simulink model "architecture_model"  (R2024a)
settings: Solver=VariableStepAuto  StartTime=0.0  StopTime=10.0  RelTol=1e-3
settings Model: Creator=nicol  LastModifiedBy=nicol

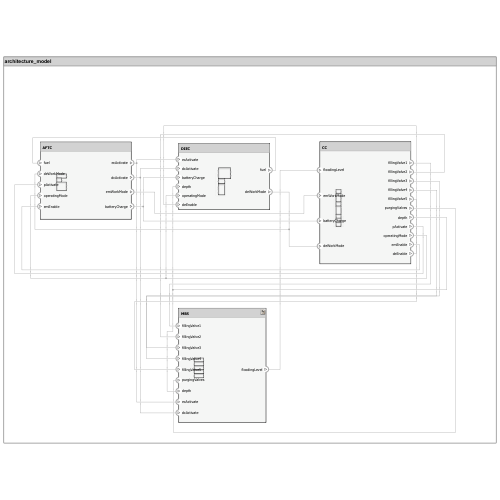
[thumbnail: Simulink's stored preview of the top-level diagram]
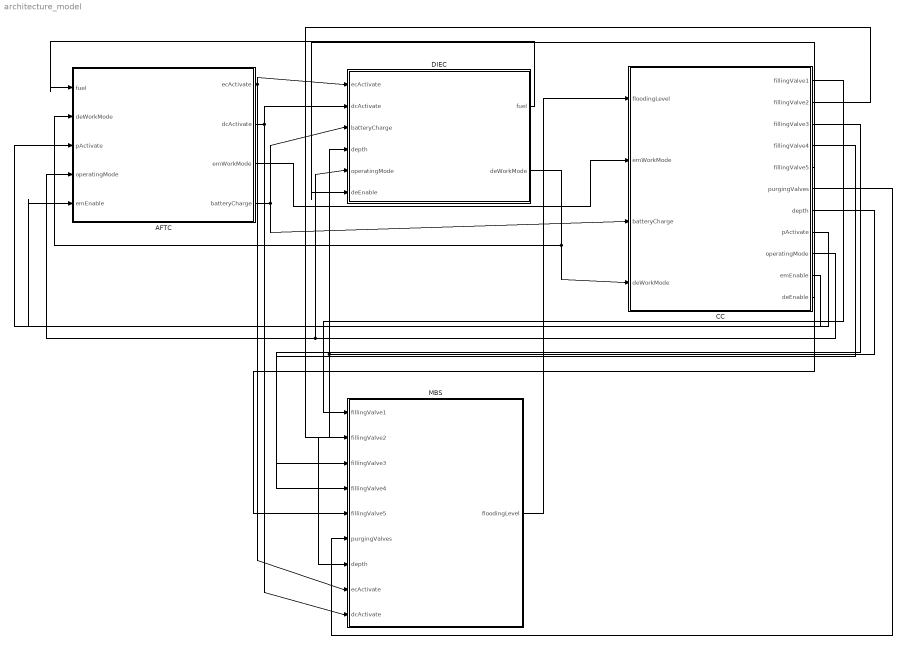
== system architecture_model ==
  AFTC : Subsystem
      settings: PortSchema="{\"entries\":[{\"content\":{\"headerSize\":26,\"margin\":15,\"minimumSpacing\":25,\"sides\":[{\"content\":{\"connectorIds\":[\"In1\",\"In2\",\"In3\",\"In4\",\"In5\"]},\"type\":\"ConnectorPlacement.EquallySpacedRectSide\",\"uuid\":\"054348e9-4623-4d1e-a130-1e3dd56bb1c6\"},{\"content\":{\"connectorIds\":[\"Out1\",\"Out2\",\"Out3\",\"Out4\"],\"side\":\"RIGHT\"},\"type\":\"ConnectorPlacement.EquallySpacedRectSide\",\"uuid\":\"04ca0bbb-2ad8-4415-8a15-39e786354471\"},{\"content\":{\"side\":\"TOP\"},\"type\":\"ConnectorPlacement.EquallySpacedRectSide\",\"uuid\":\"67b55d8f-8342-4ecc-881d-538334cee7ba\"}]},\"type\":\"ConnectorPlacement.EquallySpacedConnector\",\"uuid\":\"5f8a1871-b485-48ba-829b-ead526173e4c\"}],\"packageUris\":[\"http://schema.mathworks.com/mf0/Connector/R2020b\"],\"version\":\"1.0\"}"
  CC : Subsystem
      settings: PortSchema="{\"entries\":[{\"content\":{\"headerSize\":26,\"margin\":15,\"minimumSpacing\":25,\"sides\":[{\"content\":{\"connectorIds\":[\"In1\",\"In2\",\"In3\",\"In4\"]},\"type\":\"ConnectorPlacement.EquallySpacedRectSide\",\"uuid\":\"054348e9-4623-4d1e-a130-1e3dd56bb1c6\"},{\"content\":{\"connectorIds\":[\"Out1\",\"Out2\",\"Out3\",\"Out4\",\"Out5\",\"Out6\",\"Out7\",\"Out8\",\"Out9\",\"Out10\",\"Out11\"],\"side\":\"RIGHT\"},\"type\":\"ConnectorPlacement.EquallySpacedRectSide\",\"uuid\":\"04ca0bbb-2ad8-4415-8a15-39e786354471\"},{\"content\":{\"side\":\"TOP\"},\"type\":\"ConnectorPlacement.EquallySpacedRectSide\",\"uuid\":\"67b55d8f-8342-4ecc-881d-538334cee7ba\"}]},\"type\":\"ConnectorPlacement.EquallySpacedConnector\",\"uuid\":\"5f8a1871-b485-48ba-829b-ead526173e4c\"}],\"packageUris\":[\"http://schema.mathworks.com/mf0/Connector/R2020b\"],\"version\":\"1.0\"}"
  DIEC : Subsystem
      settings: PortSchema="{\"entries\":[{\"content\":{\"headerSize\":26,\"margin\":15,\"minimumSpacing\":25,\"sides\":[{\"content\":{\"connectorIds\":[\"In1\",\"In2\",\"In3\",\"In4\",\"In5\",\"In6\"]},\"type\":\"ConnectorPlacement.EquallySpacedRectSide\",\"uuid\":\"054348e9-4623-4d1e-a130-1e3dd56bb1c6\"},{\"content\":{\"connectorIds\":[\"Out1\",\"Out2\"],\"side\":\"RIGHT\"},\"type\":\"ConnectorPlacement.EquallySpacedRectSide\",\"uuid\":\"04ca0bbb-2ad8-4415-8a15-39e786354471\"},{\"content\":{\"side\":\"TOP\"},\"type\":\"ConnectorPlacement.EquallySpacedRectSide\",\"uuid\":\"67b55d8f-8342-4ecc-881d-538334cee7ba\"}]},\"type\":\"ConnectorPlacement.EquallySpacedConnector\",\"uuid\":\"5f8a1871-b485-48ba-829b-ead526173e4c\"}],\"packageUris\":[\"http://schema.mathworks.com/mf0/Connector/R2020b\"],\"version\":\"1.0\"}"
  MBS : Subsystem
      settings: PortSchema="{\"entries\":[{\"content\":{\"headerSize\":26,\"margin\":15,\"minimumSpacing\":25,\"sides\":[{\"content\":{\"connectorIds\":[\"In1\",\"In2\",\"In3\",\"In4\",\"In5\",\"In6\",\"In7\",\"In8\",\"In9\"]},\"type\":\"ConnectorPlacement.EquallySpacedRectSide\",\"uuid\":\"054348e9-4623-4d1e-a130-1e3dd56bb1c6\"},{\"content\":{\"connectorIds\":[\"Out1\"],\"side\":\"RIGHT\"},\"type\":\"ConnectorPlacement.EquallySpacedRectSide\",\"uuid\":\"04ca0bbb-2ad8-4415-8a15-39e786354471\"},{\"content\":{\"side\":\"TOP\"},\"type\":\"ConnectorPlacement.EquallySpacedRectSide\",\"uuid\":\"67b55d8f-8342-4ecc-881d-538334cee7ba\"}]},\"type\":\"ConnectorPlacement.EquallySpacedConnector\",\"uuid\":\"5f8a1871-b485-48ba-829b-ead526173e4c\"}],\"packageUris\":[\"http://schema.mathworks.com/mf0/Connector/R2020b\"],\"version\":\"1.0\"}"
  wires:
  AFTC/1(ecActivate) -> DIEC/1(ecActivate), MBS/8(ecActivate)
  MBS/1(floodingLevel) -> CC/1(floodingLevel)
  CC/1(fillingValve1) -> MBS/1(fillingValve1)
  CC/2(fillingValve2) -> MBS/2(fillingValve2)
  CC/3(fillingValve3) -> MBS/3(fillingValve3)
  CC/4(fillingValve4) -> MBS/4(fillingValve4)
  CC/5(fillingValve5) -> MBS/5(fillingValve5)
  CC/6(purgingValves) -> MBS/6(purgingValves)
  AFTC/2(dcActivate) -> DIEC/2(dcActivate), MBS/9(dcActivate)
  CC/7(depth) -> DIEC/4(depth), MBS/7(depth)
  DIEC/1(fuel) -> AFTC/1(fuel)
  AFTC/3(emWorkMode) -> CC/2(emWorkMode)
  AFTC/4(batteryCharge) -> DIEC/3(batteryCharge), CC/3(batteryCharge)
  DIEC/2(deWorkMode) -> AFTC/2(deWorkMode), CC/4(deWorkMode)
  CC/8(pActivate) -> AFTC/3(pActivate)
  CC/9(operatingMode) -> DIEC/5(operatingMode), AFTC/4(operatingMode)
  CC/10(emEnable) -> AFTC/5(emEnable)
  CC/11(deEnable) -> DIEC/6(deEnable)

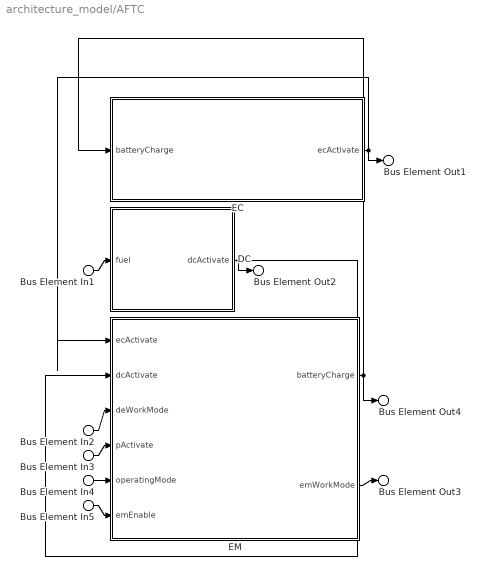
== system architecture_model/AFTC ==
  Bus Element In1 : Inport  PortName=fuel
  Bus Element In2 : Inport  Port=2  PortName=deWorkMode
  Bus Element In3 : Inport  Port=3  PortName=pActivate
  Bus Element In4 : Inport  Port=4  PortName=operatingMode
  Bus Element In5 : Inport  Port=5  PortName=emEnable
  DC : Subsystem
      settings: PortSchema="{\"entries\":[{\"content\":{\"headerSize\":26,\"margin\":15,\"minimumSpacing\":25,\"sides\":[{\"content\":{\"connectorIds\":[\"In1\"]},\"type\":\"ConnectorPlacement.EquallySpacedRectSide\",\"uuid\":\"054348e9-4623-4d1e-a130-1e3dd56bb1c6\"},{\"content\":{\"connectorIds\":[\"Out1\"],\"side\":\"RIGHT\"},\"type\":\"ConnectorPlacement.EquallySpacedRectSide\",\"uuid\":\"04ca0bbb-2ad8-4415-8a15-39e786354471\"},{\"content\":{\"side\":\"TOP\"},\"type\":\"ConnectorPlacement.EquallySpacedRectSide\",\"uuid\":\"67b55d8f-8342-4ecc-881d-538334cee7ba\"}]},\"type\":\"ConnectorPlacement.EquallySpacedConnector\",\"uuid\":\"5f8a1871-b485-48ba-829b-ead526173e4c\"}],\"packageUris\":[\"http://schema.mathworks.com/mf0/Connector/R2020b\"],\"version\":\"1.0\"}"
  EC : Subsystem
      settings: PortSchema="{\"entries\":[{\"content\":{\"headerSize\":26,\"margin\":15,\"minimumSpacing\":25,\"sides\":[{\"content\":{\"connectorIds\":[\"In1\"]},\"type\":\"ConnectorPlacement.EquallySpacedRectSide\",\"uuid\":\"054348e9-4623-4d1e-a130-1e3dd56bb1c6\"},{\"content\":{\"connectorIds\":[\"Out1\"],\"side\":\"RIGHT\"},\"type\":\"ConnectorPlacement.EquallySpacedRectSide\",\"uuid\":\"04ca0bbb-2ad8-4415-8a15-39e786354471\"},{\"content\":{\"side\":\"TOP\"},\"type\":\"ConnectorPlacement.EquallySpacedRectSide\",\"uuid\":\"67b55d8f-8342-4ecc-881d-538334cee7ba\"}]},\"type\":\"ConnectorPlacement.EquallySpacedConnector\",\"uuid\":\"5f8a1871-b485-48ba-829b-ead526173e4c\"}],\"packageUris\":[\"http://schema.mathworks.com/mf0/Connector/R2020b\"],\"version\":\"1.0\"}"
  EM : Subsystem
      settings: PortSchema="{\"entries\":[{\"content\":{\"headerSize\":26,\"margin\":15,\"minimumSpacing\":25,\"sides\":[{\"content\":{\"connectorIds\":[\"In1\",\"In2\",\"In3\",\"In4\",\"In5\",\"In6\"]},\"type\":\"ConnectorPlacement.EquallySpacedRectSide\",\"uuid\":\"054348e9-4623-4d1e-a130-1e3dd56bb1c6\"},{\"content\":{\"connectorIds\":[\"Out1\",\"Out2\"],\"side\":\"RIGHT\"},\"type\":\"ConnectorPlacement.EquallySpacedRectSide\",\"uuid\":\"04ca0bbb-2ad8-4415-8a15-39e786354471\"},{\"content\":{\"side\":\"TOP\"},\"type\":\"ConnectorPlacement.EquallySpacedRectSide\",\"uuid\":\"67b55d8f-8342-4ecc-881d-538334cee7ba\"}]},\"type\":\"ConnectorPlacement.EquallySpacedConnector\",\"uuid\":\"5f8a1871-b485-48ba-829b-ead526173e4c\"}],\"packageUris\":[\"http://schema.mathworks.com/mf0/Connector/R2020b\"],\"version\":\"1.0\"}"
  Bus Element Out1 : Outport  PortName=ecActivate
  Bus Element Out2 : Outport  Port=2  PortName=dcActivate
  Bus Element Out3 : Outport  Port=3  PortName=emWorkMode
  Bus Element Out4 : Outport  Port=4  PortName=batteryCharge
  wires:
  EC/1(ecActivate) -> Bus Element Out1/1, EM/1(ecActivate)
  EM/1(batteryCharge) -> Bus Element Out4/1, EC/1(batteryCharge)
  DC/1(dcActivate) -> Bus Element Out2/1, EM/2(dcActivate)
  Bus Element In1/1 -> DC/1(fuel)
  EM/2(emWorkMode) -> Bus Element Out3/1
  Bus Element In2/1 -> EM/3(deWorkMode)
  Bus Element In3/1 -> EM/4(pActivate)
  Bus Element In4/1 -> EM/5(operatingMode)
  Bus Element In5/1 -> EM/6(emEnable)

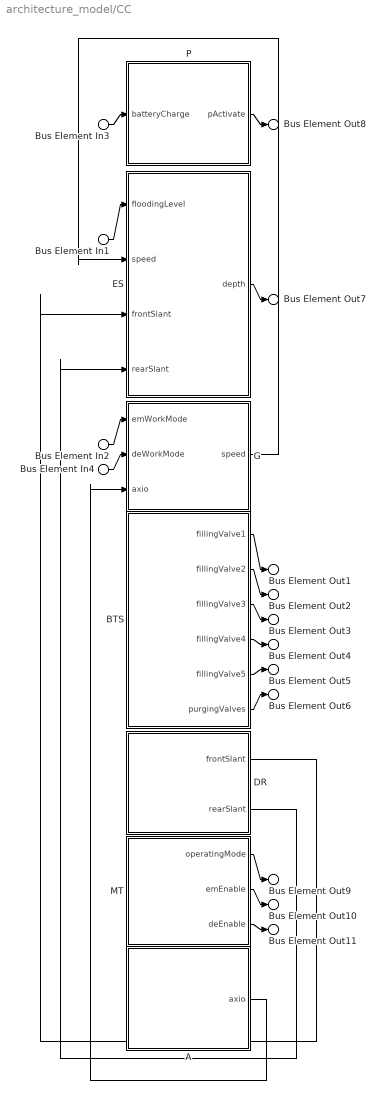
== system architecture_model/CC ==
  Bus Element In1 : Inport  PortName=floodingLevel
  Bus Element In2 : Inport  Port=2  PortName=emWorkMode
  Bus Element In3 : Inport  Port=3  PortName=batteryCharge
  Bus Element In4 : Inport  Port=4  PortName=deWorkMode
  A : Subsystem
      settings: PortSchema="{\"entries\":[{\"content\":{\"headerSize\":26,\"margin\":15,\"minimumSpacing\":25,\"sides\":[{\"content\":{},\"type\":\"ConnectorPlacement.EquallySpacedRectSide\",\"uuid\":\"054348e9-4623-4d1e-a130-1e3dd56bb1c6\"},{\"content\":{\"connectorIds\":[\"Out1\"],\"side\":\"RIGHT\"},\"type\":\"ConnectorPlacement.EquallySpacedRectSide\",\"uuid\":\"04ca0bbb-2ad8-4415-8a15-39e786354471\"},{\"content\":{\"side\":\"TOP\"},\"type\":\"ConnectorPlacement.EquallySpacedRectSide\",\"uuid\":\"67b55d8f-8342-4ecc-881d-538334cee7ba\"}]},\"type\":\"ConnectorPlacement.EquallySpacedConnector\",\"uuid\":\"5f8a1871-b485-48ba-829b-ead526173e4c\"}],\"packageUris\":[\"http://schema.mathworks.com/mf0/Connector/R2020b\"],\"version\":\"1.0\"}"
  BTS : Subsystem
      settings: PortSchema="{\"entries\":[{\"content\":{\"headerSize\":26,\"margin\":15,\"minimumSpacing\":25,\"sides\":[{\"content\":{},\"type\":\"ConnectorPlacement.EquallySpacedRectSide\",\"uuid\":\"054348e9-4623-4d1e-a130-1e3dd56bb1c6\"},{\"content\":{\"connectorIds\":[\"Out1\",\"Out2\",\"Out3\",\"Out4\",\"Out5\",\"Out6\"],\"side\":\"RIGHT\"},\"type\":\"ConnectorPlacement.EquallySpacedRectSide\",\"uuid\":\"04ca0bbb-2ad8-4415-8a15-39e786354471\"},{\"content\":{\"side\":\"TOP\"},\"type\":\"ConnectorPlacement.EquallySpacedRectSide\",\"uuid\":\"67b55d8f-8342-4ecc-881d-538334cee7ba\"}]},\"type\":\"ConnectorPlacement.EquallySpacedConnector\",\"uuid\":\"5f8a1871-b485-48ba-829b-ead526173e4c\"}],\"packageUris\":[\"http://schema.mathworks.com/mf0/Connector/R2020b\"],\"version\":\"1.0\"}"
  DR : Subsystem
      settings: PortSchema="{\"entries\":[{\"content\":{\"headerSize\":26,\"margin\":15,\"minimumSpacing\":25,\"sides\":[{\"content\":{},\"type\":\"ConnectorPlacement.EquallySpacedRectSide\",\"uuid\":\"054348e9-4623-4d1e-a130-1e3dd56bb1c6\"},{\"content\":{\"connectorIds\":[\"Out1\",\"Out2\"],\"side\":\"RIGHT\"},\"type\":\"ConnectorPlacement.EquallySpacedRectSide\",\"uuid\":\"04ca0bbb-2ad8-4415-8a15-39e786354471\"},{\"content\":{\"side\":\"TOP\"},\"type\":\"ConnectorPlacement.EquallySpacedRectSide\",\"uuid\":\"67b55d8f-8342-4ecc-881d-538334cee7ba\"}]},\"type\":\"ConnectorPlacement.EquallySpacedConnector\",\"uuid\":\"5f8a1871-b485-48ba-829b-ead526173e4c\"}],\"packageUris\":[\"http://schema.mathworks.com/mf0/Connector/R2020b\"],\"version\":\"1.0\"}"
  ES : Subsystem
      settings: PortSchema="{\"entries\":[{\"content\":{\"headerSize\":26,\"margin\":15,\"minimumSpacing\":25,\"sides\":[{\"content\":{\"connectorIds\":[\"In1\",\"In2\",\"In3\",\"In4\"]},\"type\":\"ConnectorPlacement.EquallySpacedRectSide\",\"uuid\":\"054348e9-4623-4d1e-a130-1e3dd56bb1c6\"},{\"content\":{\"connectorIds\":[\"Out1\"],\"side\":\"RIGHT\"},\"type\":\"ConnectorPlacement.EquallySpacedRectSide\",\"uuid\":\"04ca0bbb-2ad8-4415-8a15-39e786354471\"},{\"content\":{\"side\":\"TOP\"},\"type\":\"ConnectorPlacement.EquallySpacedRectSide\",\"uuid\":\"67b55d8f-8342-4ecc-881d-538334cee7ba\"}]},\"type\":\"ConnectorPlacement.EquallySpacedConnector\",\"uuid\":\"5f8a1871-b485-48ba-829b-ead526173e4c\"}],\"packageUris\":[\"http://schema.mathworks.com/mf0/Connector/R2020b\"],\"version\":\"1.0\"}"
  G : Subsystem
      settings: PortSchema="{\"entries\":[{\"content\":{\"headerSize\":26,\"margin\":15,\"minimumSpacing\":25,\"sides\":[{\"content\":{\"connectorIds\":[\"In1\",\"In2\",\"In3\"]},\"type\":\"ConnectorPlacement.EquallySpacedRectSide\",\"uuid\":\"054348e9-4623-4d1e-a130-1e3dd56bb1c6\"},{\"content\":{\"connectorIds\":[\"Out1\"],\"side\":\"RIGHT\"},\"type\":\"ConnectorPlacement.EquallySpacedRectSide\",\"uuid\":\"04ca0bbb-2ad8-4415-8a15-39e786354471\"},{\"content\":{\"side\":\"TOP\"},\"type\":\"ConnectorPlacement.EquallySpacedRectSide\",\"uuid\":\"67b55d8f-8342-4ecc-881d-538334cee7ba\"}]},\"type\":\"ConnectorPlacement.EquallySpacedConnector\",\"uuid\":\"5f8a1871-b485-48ba-829b-ead526173e4c\"}],\"packageUris\":[\"http://schema.mathworks.com/mf0/Connector/R2020b\"],\"version\":\"1.0\"}"
  MT : Subsystem
      settings: PortSchema="{\"entries\":[{\"content\":{\"headerSize\":26,\"margin\":15,\"minimumSpacing\":25,\"sides\":[{\"content\":{},\"type\":\"ConnectorPlacement.EquallySpacedRectSide\",\"uuid\":\"054348e9-4623-4d1e-a130-1e3dd56bb1c6\"},{\"content\":{\"connectorIds\":[\"Out1\",\"Out2\",\"Out3\"],\"side\":\"RIGHT\"},\"type\":\"ConnectorPlacement.EquallySpacedRectSide\",\"uuid\":\"04ca0bbb-2ad8-4415-8a15-39e786354471\"},{\"content\":{\"side\":\"TOP\"},\"type\":\"ConnectorPlacement.EquallySpacedRectSide\",\"uuid\":\"67b55d8f-8342-4ecc-881d-538334cee7ba\"}]},\"type\":\"ConnectorPlacement.EquallySpacedConnector\",\"uuid\":\"5f8a1871-b485-48ba-829b-ead526173e4c\"}],\"packageUris\":[\"http://schema.mathworks.com/mf0/Connector/R2020b\"],\"version\":\"1.0\"}"
  P : Subsystem
      settings: PortSchema="{\"entries\":[{\"content\":{\"headerSize\":26,\"margin\":15,\"minimumSpacing\":25,\"sides\":[{\"content\":{\"connectorIds\":[\"In1\"]},\"type\":\"ConnectorPlacement.EquallySpacedRectSide\",\"uuid\":\"054348e9-4623-4d1e-a130-1e3dd56bb1c6\"},{\"content\":{\"connectorIds\":[\"Out1\"],\"side\":\"RIGHT\"},\"type\":\"ConnectorPlacement.EquallySpacedRectSide\",\"uuid\":\"04ca0bbb-2ad8-4415-8a15-39e786354471\"},{\"content\":{\"side\":\"TOP\"},\"type\":\"ConnectorPlacement.EquallySpacedRectSide\",\"uuid\":\"67b55d8f-8342-4ecc-881d-538334cee7ba\"}]},\"type\":\"ConnectorPlacement.EquallySpacedConnector\",\"uuid\":\"5f8a1871-b485-48ba-829b-ead526173e4c\"}],\"packageUris\":[\"http://schema.mathworks.com/mf0/Connector/R2020b\"],\"version\":\"1.0\"}"
  Bus Element Out1 : Outport  PortName=fillingValve1
  Bus Element Out2 : Outport  Port=2  PortName=fillingValve2
  Bus Element Out3 : Outport  Port=3  PortName=fillingValve3
  Bus Element Out4 : Outport  Port=4  PortName=fillingValve4
  Bus Element Out5 : Outport  Port=5  PortName=fillingValve5
  Bus Element Out6 : Outport  Port=6  PortName=purgingValves
  Bus Element Out7 : Outport  Port=7  PortName=depth
  Bus Element Out8 : Outport  Port=8  PortName=pActivate
  Bus Element Out9 : Outport  Port=9  PortName=operatingMode
  Bus Element Out10 : Outport  Port=10  PortName=emEnable
  Bus Element Out11 : Outport  Port=11  PortName=deEnable
  wires:
  Bus Element In1/1 -> ES/1(floodingLevel)
  BTS/1(fillingValve1) -> Bus Element Out1/1
  BTS/2(fillingValve2) -> Bus Element Out2/1
  BTS/3(fillingValve3) -> Bus Element Out3/1
  BTS/4(fillingValve4) -> Bus Element Out4/1
  BTS/5(fillingValve5) -> Bus Element Out5/1
  BTS/6(purgingValves) -> Bus Element Out6/1
  ES/1(depth) -> Bus Element Out7/1
  Bus Element In2/1 -> G/1(emWorkMode)
  Bus Element In3/1 -> P/1(batteryCharge)
  P/1(pActivate) -> Bus Element Out8/1
  MT/1(operatingMode) -> Bus Element Out9/1
  MT/2(emEnable) -> Bus Element Out10/1
  Bus Element In4/1 -> G/2(deWorkMode)
  G/1(speed) -> ES/2(speed)
  DR/1(frontSlant) -> ES/3(frontSlant)
  DR/2(rearSlant) -> ES/4(rearSlant)
  A/1(axio) -> G/3(axio)
  MT/3(deEnable) -> Bus Element Out11/1

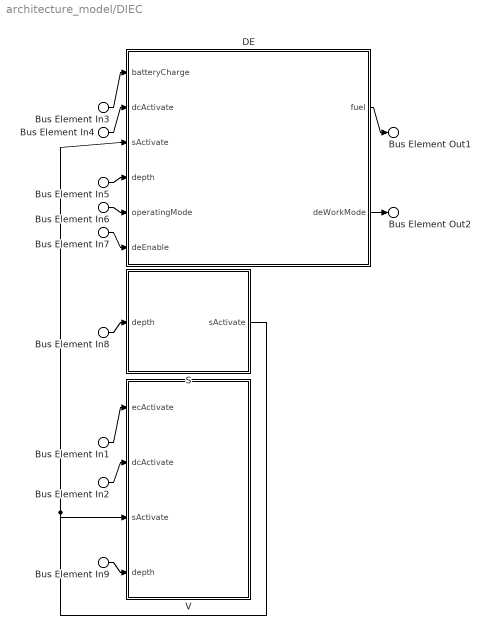
== system architecture_model/DIEC ==
  Bus Element In1 : Inport  PortName=ecActivate
  Bus Element In2 : Inport  Port=2  PortName=dcActivate
  Bus Element In4 : Inport  Port=2  PortName=dcActivate
  Bus Element In3 : Inport  Port=3  PortName=batteryCharge
  Bus Element In5 : Inport  Port=4  PortName=depth
  Bus Element In8 : Inport  Port=4  PortName=depth
  Bus Element In9 : Inport  Port=4  PortName=depth
  Bus Element In6 : Inport  Port=5  PortName=operatingMode
  Bus Element In7 : Inport  Port=6  PortName=deEnable
  DE : Subsystem
      settings: PortSchema="{\"entries\":[{\"content\":{\"headerSize\":26,\"margin\":15,\"minimumSpacing\":25,\"sides\":[{\"content\":{\"connectorIds\":[\"In1\",\"In2\",\"In3\",\"In4\",\"In5\",\"In6\"]},\"type\":\"ConnectorPlacement.EquallySpacedRectSide\",\"uuid\":\"054348e9-4623-4d1e-a130-1e3dd56bb1c6\"},{\"content\":{\"connectorIds\":[\"Out1\",\"Out2\"],\"side\":\"RIGHT\"},\"type\":\"ConnectorPlacement.EquallySpacedRectSide\",\"uuid\":\"04ca0bbb-2ad8-4415-8a15-39e786354471\"},{\"content\":{\"side\":\"TOP\"},\"type\":\"ConnectorPlacement.EquallySpacedRectSide\",\"uuid\":\"67b55d8f-8342-4ecc-881d-538334cee7ba\"}]},\"type\":\"ConnectorPlacement.EquallySpacedConnector\",\"uuid\":\"5f8a1871-b485-48ba-829b-ead526173e4c\"}],\"packageUris\":[\"http://schema.mathworks.com/mf0/Connector/R2020b\"],\"version\":\"1.0\"}"
  S : Subsystem
      settings: PortSchema="{\"entries\":[{\"content\":{\"headerSize\":26,\"margin\":15,\"minimumSpacing\":25,\"sides\":[{\"content\":{\"connectorIds\":[\"In1\"]},\"type\":\"ConnectorPlacement.EquallySpacedRectSide\",\"uuid\":\"054348e9-4623-4d1e-a130-1e3dd56bb1c6\"},{\"content\":{\"connectorIds\":[\"Out1\"],\"side\":\"RIGHT\"},\"type\":\"ConnectorPlacement.EquallySpacedRectSide\",\"uuid\":\"04ca0bbb-2ad8-4415-8a15-39e786354471\"},{\"content\":{\"side\":\"TOP\"},\"type\":\"ConnectorPlacement.EquallySpacedRectSide\",\"uuid\":\"67b55d8f-8342-4ecc-881d-538334cee7ba\"}]},\"type\":\"ConnectorPlacement.EquallySpacedConnector\",\"uuid\":\"5f8a1871-b485-48ba-829b-ead526173e4c\"}],\"packageUris\":[\"http://schema.mathworks.com/mf0/Connector/R2020b\"],\"version\":\"1.0\"}"
  V : Subsystem
      settings: PortSchema="{\"entries\":[{\"content\":{\"headerSize\":26,\"margin\":15,\"minimumSpacing\":25,\"sides\":[{\"content\":{\"connectorIds\":[\"In1\",\"In2\",\"In3\",\"In4\"]},\"type\":\"ConnectorPlacement.EquallySpacedRectSide\",\"uuid\":\"054348e9-4623-4d1e-a130-1e3dd56bb1c6\"},{\"content\":{\"side\":\"RIGHT\"},\"type\":\"ConnectorPlacement.EquallySpacedRectSide\",\"uuid\":\"04ca0bbb-2ad8-4415-8a15-39e786354471\"},{\"content\":{\"side\":\"TOP\"},\"type\":\"ConnectorPlacement.EquallySpacedRectSide\",\"uuid\":\"67b55d8f-8342-4ecc-881d-538334cee7ba\"}]},\"type\":\"ConnectorPlacement.EquallySpacedConnector\",\"uuid\":\"5f8a1871-b485-48ba-829b-ead526173e4c\"}],\"packageUris\":[\"http://schema.mathworks.com/mf0/Connector/R2020b\"],\"version\":\"1.0\"}"
  Bus Element Out1 : Outport  PortName=fuel
  Bus Element Out2 : Outport  Port=2  PortName=deWorkMode
  wires:
  Bus Element In1/1 -> V/1(ecActivate)
  Bus Element In2/1 -> V/2(dcActivate)
  Bus Element In3/1 -> DE/1(batteryCharge)
  DE/2(deWorkMode) -> Bus Element Out2/1
  DE/1(fuel) -> Bus Element Out1/1
  Bus Element In4/1 -> DE/2(dcActivate)
  S/1(sActivate) -> DE/3(sActivate), V/3(sActivate)
  Bus Element In5/1 -> DE/4(depth)
  Bus Element In6/1 -> DE/5(operatingMode)
  Bus Element In7/1 -> DE/6(deEnable)
  Bus Element In8/1 -> S/1(depth)
  Bus Element In9/1 -> V/4(depth)

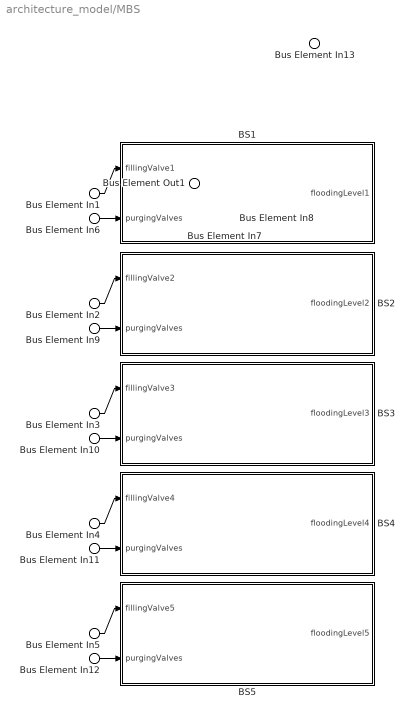
== system architecture_model/MBS ==
  Bus Element In1 : Inport  PortName=fillingValve1
  Bus Element In2 : Inport  Port=2  PortName=fillingValve2
  Bus Element In3 : Inport  Port=3  PortName=fillingValve3
  Bus Element In4 : Inport  Port=4  PortName=fillingValve4
  Bus Element In5 : Inport  Port=5  PortName=fillingValve5
  Bus Element In{6,9..12} (5 alike) : Inport  Port=6  PortName=purgingValves
  Bus Element In13 : Inport  Port=7  PortName=depth
  Bus Element In7 : Inport  Port=8  PortName=ecActivate
  Bus Element In8 : Inport  Port=9  PortName=dcActivate
  BS1 : Subsystem
      settings: PortSchema="{\"entries\":[{\"content\":{\"headerSize\":26,\"margin\":15,\"minimumSpacing\":25,\"sides\":[{\"content\":{\"connectorIds\":[\"In1\",\"In2\"]},\"type\":\"ConnectorPlacement.EquallySpacedRectSide\",\"uuid\":\"054348e9-4623-4d1e-a130-1e3dd56bb1c6\"},{\"content\":{\"connectorIds\":[\"Out1\"],\"side\":\"RIGHT\"},\"type\":\"ConnectorPlacement.EquallySpacedRectSide\",\"uuid\":\"04ca0bbb-2ad8-4415-8a15-39e786354471\"},{\"content\":{\"side\":\"TOP\"},\"type\":\"ConnectorPlacement.EquallySpacedRectSide\",\"uuid\":\"67b55d8f-8342-4ecc-881d-538334cee7ba\"}]},\"type\":\"ConnectorPlacement.EquallySpacedConnector\",\"uuid\":\"5f8a1871-b485-48ba-829b-ead526173e4c\"}],\"packageUris\":[\"http://schema.mathworks.com/mf0/Connector/R2020b\"],\"version\":\"1.0\"}"
  BS2 : Subsystem
      settings: PortSchema="{\"entries\":[{\"content\":{\"headerSize\":26,\"margin\":15,\"minimumSpacing\":25,\"sides\":[{\"content\":{\"connectorIds\":[\"In1\",\"In2\"]},\"type\":\"ConnectorPlacement.EquallySpacedRectSide\",\"uuid\":\"054348e9-4623-4d1e-a130-1e3dd56bb1c6\"},{\"content\":{\"connectorIds\":[\"Out1\"],\"side\":\"RIGHT\"},\"type\":\"ConnectorPlacement.EquallySpacedRectSide\",\"uuid\":\"04ca0bbb-2ad8-4415-8a15-39e786354471\"},{\"content\":{\"side\":\"TOP\"},\"type\":\"ConnectorPlacement.EquallySpacedRectSide\",\"uuid\":\"67b55d8f-8342-4ecc-881d-538334cee7ba\"}]},\"type\":\"ConnectorPlacement.EquallySpacedConnector\",\"uuid\":\"5f8a1871-b485-48ba-829b-ead526173e4c\"}],\"packageUris\":[\"http://schema.mathworks.com/mf0/Connector/R2020b\"],\"version\":\"1.0\"}"
  BS3 : Subsystem
      settings: PortSchema="{\"entries\":[{\"content\":{\"headerSize\":26,\"margin\":15,\"minimumSpacing\":25,\"sides\":[{\"content\":{\"connectorIds\":[\"In1\",\"In2\"]},\"type\":\"ConnectorPlacement.EquallySpacedRectSide\",\"uuid\":\"054348e9-4623-4d1e-a130-1e3dd56bb1c6\"},{\"content\":{\"connectorIds\":[\"Out1\"],\"side\":\"RIGHT\"},\"type\":\"ConnectorPlacement.EquallySpacedRectSide\",\"uuid\":\"04ca0bbb-2ad8-4415-8a15-39e786354471\"},{\"content\":{\"side\":\"TOP\"},\"type\":\"ConnectorPlacement.EquallySpacedRectSide\",\"uuid\":\"67b55d8f-8342-4ecc-881d-538334cee7ba\"}]},\"type\":\"ConnectorPlacement.EquallySpacedConnector\",\"uuid\":\"5f8a1871-b485-48ba-829b-ead526173e4c\"}],\"packageUris\":[\"http://schema.mathworks.com/mf0/Connector/R2020b\"],\"version\":\"1.0\"}"
  BS4 : Subsystem
      settings: PortSchema="{\"entries\":[{\"content\":{\"headerSize\":26,\"margin\":15,\"minimumSpacing\":25,\"sides\":[{\"content\":{\"connectorIds\":[\"In1\",\"In2\"]},\"type\":\"ConnectorPlacement.EquallySpacedRectSide\",\"uuid\":\"054348e9-4623-4d1e-a130-1e3dd56bb1c6\"},{\"content\":{\"connectorIds\":[\"Out1\"],\"side\":\"RIGHT\"},\"type\":\"ConnectorPlacement.EquallySpacedRectSide\",\"uuid\":\"04ca0bbb-2ad8-4415-8a15-39e786354471\"},{\"content\":{\"side\":\"TOP\"},\"type\":\"ConnectorPlacement.EquallySpacedRectSide\",\"uuid\":\"67b55d8f-8342-4ecc-881d-538334cee7ba\"}]},\"type\":\"ConnectorPlacement.EquallySpacedConnector\",\"uuid\":\"5f8a1871-b485-48ba-829b-ead526173e4c\"}],\"packageUris\":[\"http://schema.mathworks.com/mf0/Connector/R2020b\"],\"version\":\"1.0\"}"
  BS5 : Subsystem
      settings: PortSchema="{\"entries\":[{\"content\":{\"headerSize\":26,\"margin\":15,\"minimumSpacing\":25,\"sides\":[{\"content\":{\"connectorIds\":[\"In1\",\"In2\"]},\"type\":\"ConnectorPlacement.EquallySpacedRectSide\",\"uuid\":\"054348e9-4623-4d1e-a130-1e3dd56bb1c6\"},{\"content\":{\"connectorIds\":[\"Out1\"],\"side\":\"RIGHT\"},\"type\":\"ConnectorPlacement.EquallySpacedRectSide\",\"uuid\":\"04ca0bbb-2ad8-4415-8a15-39e786354471\"},{\"content\":{\"side\":\"TOP\"},\"type\":\"ConnectorPlacement.EquallySpacedRectSide\",\"uuid\":\"67b55d8f-8342-4ecc-881d-538334cee7ba\"}]},\"type\":\"ConnectorPlacement.EquallySpacedConnector\",\"uuid\":\"5f8a1871-b485-48ba-829b-ead526173e4c\"}],\"packageUris\":[\"http://schema.mathworks.com/mf0/Connector/R2020b\"],\"version\":\"1.0\"}"
  Bus Element Out1 : Outport  PortName=floodingLevel
  wires:
  Bus Element In1/1 -> BS1/1(fillingValve1)
  Bus Element In2/1 -> BS2/1(fillingValve2)
  Bus Element In3/1 -> BS3/1(fillingValve3)
  Bus Element In4/1 -> BS4/1(fillingValve4)
  Bus Element In5/1 -> BS5/1(fillingValve5)
  Bus Element In6/1 -> BS1/2(purgingValves)
  Bus Element In9/1 -> BS2/2(purgingValves)
  Bus Element In10/1 -> BS3/2(purgingValves)
  Bus Element In11/1 -> BS4/2(purgingValves)
  Bus Element In12/1 -> BS5/2(purgingValves)

== system architecture_model/AFTC/DC ==
  Bus Element In1 : Inport  PortName=fuel
  Bus Element Out1 : Outport  PortName=dcActivate

== system architecture_model/AFTC/EC ==
  Bus Element In1 : Inport  PortName=batteryCharge
  Bus Element Out1 : Outport  PortName=ecActivate

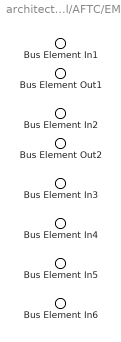
== system architecture_model/AFTC/EM ==
  Bus Element In1 : Inport  PortName=ecActivate
  Bus Element In2 : Inport  Port=2  PortName=dcActivate
  Bus Element In3 : Inport  Port=3  PortName=deWorkMode
  Bus Element In4 : Inport  Port=4  PortName=pActivate
  Bus Element In5 : Inport  Port=5  PortName=operatingMode
  Bus Element In6 : Inport  Port=6  PortName=emEnable
  Bus Element Out1 : Outport  PortName=batteryCharge
  Bus Element Out2 : Outport  Port=2  PortName=emWorkMode

== system architecture_model/CC/A ==
  Bus Element Out1 : Outport  PortName=axio

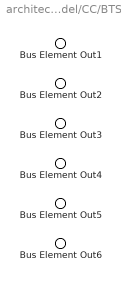
== system architecture_model/CC/BTS ==
  Bus Element Out1 : Outport  PortName=fillingValve1
  Bus Element Out2 : Outport  Port=2  PortName=fillingValve2
  Bus Element Out3 : Outport  Port=3  PortName=fillingValve3
  Bus Element Out4 : Outport  Port=4  PortName=fillingValve4
  Bus Element Out5 : Outport  Port=5  PortName=fillingValve5
  Bus Element Out6 : Outport  Port=6  PortName=purgingValves

== system architecture_model/CC/DR ==
  Bus Element Out1 : Outport  PortName=frontSlant
  Bus Element Out2 : Outport  Port=2  PortName=rearSlant

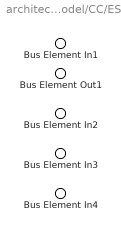
== system architecture_model/CC/ES ==
  Bus Element In1 : Inport  PortName=floodingLevel
  Bus Element In2 : Inport  Port=2  PortName=speed
  Bus Element In3 : Inport  Port=3  PortName=frontSlant
  Bus Element In4 : Inport  Port=4  PortName=rearSlant
  Bus Element Out1 : Outport  PortName=depth

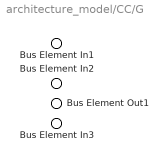
== system architecture_model/CC/G ==
  Bus Element In1 : Inport  PortName=emWorkMode
  Bus Element In2 : Inport  Port=2  PortName=deWorkMode
  Bus Element In3 : Inport  Port=3  PortName=axio
  Bus Element Out1 : Outport  PortName=speed

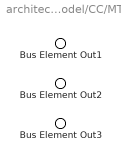
== system architecture_model/CC/MT ==
  Bus Element Out1 : Outport  PortName=operatingMode
  Bus Element Out2 : Outport  Port=2  PortName=emEnable
  Bus Element Out3 : Outport  Port=3  PortName=deEnable

== system architecture_model/CC/P ==
  Bus Element In1 : Inport  PortName=batteryCharge
  Bus Element Out1 : Outport  PortName=pActivate

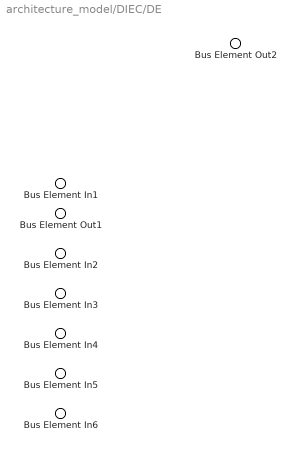
== system architecture_model/DIEC/DE ==
  Bus Element In1 : Inport  PortName=batteryCharge
  Bus Element In2 : Inport  Port=2  PortName=dcActivate
  Bus Element In3 : Inport  Port=3  PortName=sActivate
  Bus Element In4 : Inport  Port=4  PortName=depth
  Bus Element In5 : Inport  Port=5  PortName=operatingMode
  Bus Element In6 : Inport  Port=6  PortName=deEnable
  Bus Element Out2 : Outport  PortName=fuel
  Bus Element Out1 : Outport  Port=2  PortName=deWorkMode

== system architecture_model/DIEC/S ==
  Bus Element In1 : Inport  PortName=depth
  Bus Element Out1 : Outport  PortName=sActivate

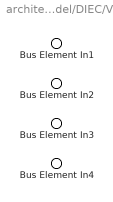
== system architecture_model/DIEC/V ==
  Bus Element In1 : Inport  PortName=ecActivate
  Bus Element In2 : Inport  Port=2  PortName=dcActivate
  Bus Element In3 : Inport  Port=3  PortName=sActivate
  Bus Element In4 : Inport  Port=4  PortName=depth

== system architecture_model/MBS/BS1 ==
  Bus Element In1 : Inport  PortName=fillingValve1
  Bus Element In2 : Inport  Port=2  PortName=purgingValves
  Bus Element Out1 : Outport  PortName=floodingLevel1

== system architecture_model/MBS/BS2 ==
  Bus Element In1 : Inport  PortName=fillingValve2
  Bus Element In2 : Inport  Port=2  PortName=purgingValves
  Bus Element Out1 : Outport  PortName=floodingLevel2

== system architecture_model/MBS/BS3 ==
  Bus Element In1 : Inport  PortName=fillingValve3
  Bus Element In2 : Inport  Port=2  PortName=purgingValves
  Bus Element Out1 : Outport  PortName=floodingLevel3

== system architecture_model/MBS/BS4 ==
  Bus Element In1 : Inport  PortName=fillingValve4
  Bus Element In2 : Inport  Port=2  PortName=purgingValves
  Bus Element Out1 : Outport  PortName=floodingLevel4

== system architecture_model/MBS/BS5 ==
  Bus Element In1 : Inport  PortName=fillingValve5
  Bus Element In2 : Inport  Port=2  PortName=purgingValves
  Bus Element Out1 : Outport  PortName=floodingLevel5
